simulink model "prob5"  (R2013a)
settings: Solver=ode45  StartTime=0.0  StopTime=5  RelTol=1e-3
libraries: simulink x1
settings Model: Creator=Suddenlink  LastModifiedBy=Suddenlink

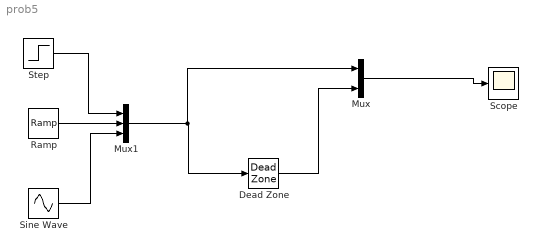
== system prob5 ==
  Dead Zone : DeadZone  SaturateOnIntegerOverflow=on
  Mux : Mux  Inputs=2
  Mux1 : Mux  Inputs=3
  Ramp : simulink/Sources/Ramp  slope=1  start=0  X0=0
  Scope : Scope
      settings: TimeRange=5
  Sine Wave : Sin  Amplitude=5  Frequency=2*pi  SampleTime=0
  Step : Step  After=5  SampleTime=0
  wires:
  Mux/1 -> Scope/1
  Dead Zone/1 -> Mux/2
  Mux1/1 -> Mux/1, Dead Zone/1
  Step/1 -> Mux1/1
  Ramp/1 -> Mux1/2
  Sine Wave/1 -> Mux1/3
